simulink model "spacecraft_adcs"  (R2025b)
settings: Solver=ode4  StartTime=0.0  StopTime=600  FixedStep=0.01  RelTol=1e-3
InitFcn:
  | init_spacecraft_adcs
values from neighbouring files (symbols this model uses):
  mekf_params = struct()    [init_spacecraft_adcs.m]
undefined symbols (not defined in the file or in its folder): env, init, orbit, ref_time, sensors, sim_params, spacecraft
settings Model: Creator=cutcu  LastModifiedBy=cutcu

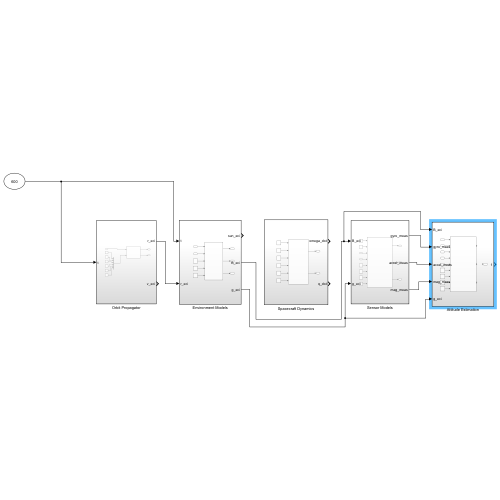
[thumbnail: Simulink's stored preview of the top-level diagram]
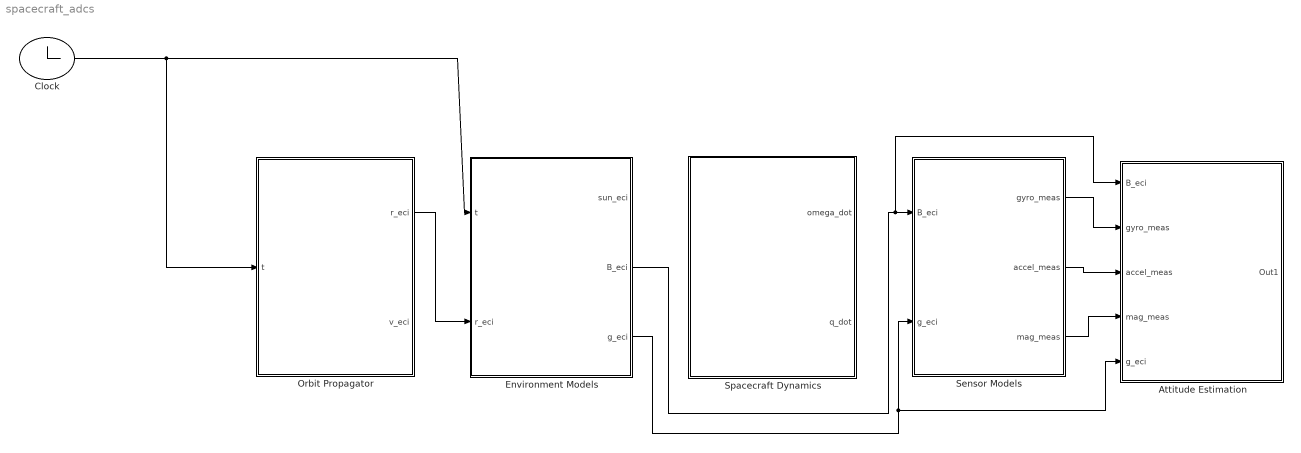
== system spacecraft_adcs ==
  Attitude Estimation : Subsystem
  Clock : Clock
  Environment Models : Subsystem
  Orbit Propagator : Subsystem
  Sensor Models : Subsystem
  Spacecraft Dynamics : Subsystem
  wires:
  Orbit Propagator/1(r_eci) -> Environment Models/2(r_eci)
  Clock/1 -> Environment Models/1(t), Orbit Propagator/1(t)
  Environment Models/3(g_eci) -> Attitude Estimation/5(g_eci), Sensor Models/2(g_eci)
  Environment Models/2(B_eci) -> Attitude Estimation/1(B_eci), Sensor Models/1(B_eci)
  Sensor Models/1(gyro_meas) -> Attitude Estimation/2(gyro_meas)
  Sensor Models/2(accel_meas) -> Attitude Estimation/3(accel_meas)
  Sensor Models/3(mag_meas) -> Attitude Estimation/4(mag_meas)

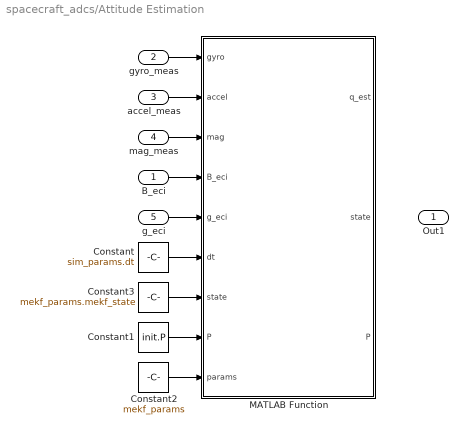
== system spacecraft_adcs/Attitude Estimation ==
  B_eci : Inport
  gyro_meas : Inport  Port=2
  accel_meas : Inport  Port=3
  mag_meas : Inport  Port=4
  g_eci : Inport  Port=5
  Constant : Constant  Value=sim_params.dt
  Constant1 : Constant  Value=init.P
  Constant2 : Constant  Value=mekf_params
  Constant3 : Constant  Value=mekf_params.mekf_state
  MATLAB Function : MATLAB Function  TreatAsAtomicUnit=on
  Out1 : Outport
  wires:
  gyro_meas/1 -> MATLAB Function/1(gyro)
  accel_meas/1 -> MATLAB Function/2(accel)
  mag_meas/1 -> MATLAB Function/3(mag)
  Constant/1 -> MATLAB Function/6(dt)
  Constant1/1 -> MATLAB Function/8("P ")
  Constant2/1 -> MATLAB Function/9(params)
  Constant3/1 -> MATLAB Function/7("state ")
  g_eci/1 -> MATLAB Function/5(g_eci)
  B_eci/1 -> MATLAB Function/4(B_eci)

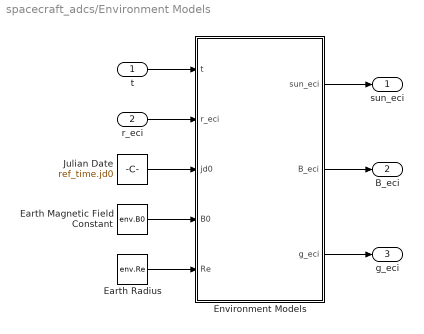
== system spacecraft_adcs/Environment Models ==
  t : Inport
  r_eci : Inport  Port=2
  Earth Magnetic Field Constant : Constant  Value=env.B0
  Earth Radius : Constant  Value=env.Re
  Environment Models : MATLAB Function  TreatAsAtomicUnit=on
  Julian Date : Constant  Value=ref_time.jd0
  sun_eci : Outport
  B_eci : Outport  Port=2
  g_eci : Outport  Port=3
  wires:
  r_eci/1 -> Environment Models/2(r_eci)
  Julian Date/1 -> Environment Models/3(jd0)
  Earth Magnetic Field Constant/1 -> Environment Models/4(B0)
  Earth Radius/1 -> Environment Models/5(Re)
  Environment Models/1(sun_eci) -> sun_eci/1
  Environment Models/2(B_eci) -> B_eci/1
  Environment Models/3(g_eci) -> g_eci/1
  t/1 -> Environment Models/1(t)

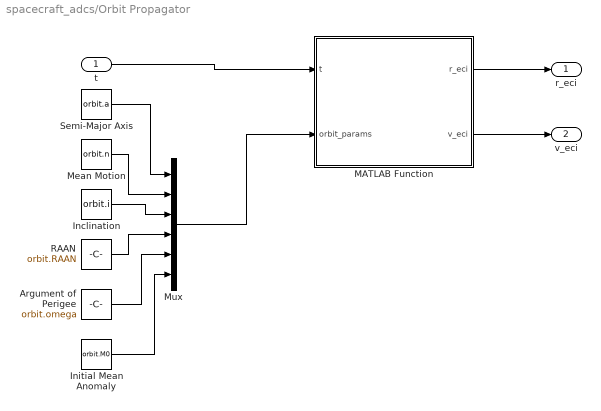
== system spacecraft_adcs/Orbit Propagator ==
  t : Inport
  Argument of Perigee : Constant  Value=orbit.omega
  Inclination : Constant  Value=orbit.i
  Initial Mean Anomaly : Constant  Value=orbit.M0
  MATLAB Function : MATLAB Function  TreatAsAtomicUnit=on
  Mean Motion : Constant  Value=orbit.n
  Mux : Mux  Inputs=6
  RAAN : Constant  Value=orbit.RAAN
  Semi-Major Axis : Constant  Value=orbit.a
  r_eci : Outport
  v_eci : Outport  Port=2
  wires:
  MATLAB Function/2(v_eci) -> v_eci/1
  MATLAB Function/1(r_eci) -> r_eci/1
  Semi-Major Axis/1 -> Mux/1
  Mean Motion/1 -> Mux/2
  Inclination/1 -> Mux/3
  RAAN/1 -> Mux/4
  Argument of Perigee/1 -> Mux/5
  Initial Mean Anomaly/1 -> Mux/6
  Mux/1 -> MATLAB Function/2(orbit_params)
  t/1 -> MATLAB Function/1(t)

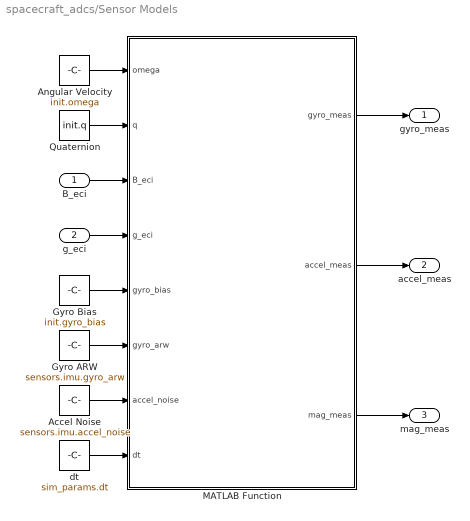
== system spacecraft_adcs/Sensor Models ==
  B_eci : Inport
  g_eci : Inport  Port=2
  Accel Noise : Constant  Value=sensors.imu.accel_noise
  Angular Velocity : Constant  Value=init.omega
  Gyro ARW : Constant  Value=sensors.imu.gyro_arw
  Gyro Bias : Constant  Value=init.gyro_bias
  MATLAB Function : MATLAB Function  TreatAsAtomicUnit=on
  Quaternion : Constant  Value=init.q
  dt : Constant  Value=sim_params.dt
  gyro_meas : Outport
  accel_meas : Outport  Port=2
  mag_meas : Outport  Port=3
  wires:
  dt/1 -> MATLAB Function/8(dt)
  B_eci/1 -> MATLAB Function/3(B_eci)
  g_eci/1 -> MATLAB Function/4(g_eci)
  Gyro ARW/1 -> MATLAB Function/6(gyro_arw)
  Accel Noise/1 -> MATLAB Function/7(accel_noise)
  Gyro Bias/1 -> MATLAB Function/5(gyro_bias)
  Quaternion/1 -> MATLAB Function/2(q)
  Angular Velocity/1 -> MATLAB Function/1(omega)
  MATLAB Function/1(gyro_meas) -> gyro_meas/1
  MATLAB Function/2(accel_meas) -> accel_meas/1
  MATLAB Function/3(mag_meas) -> mag_meas/1

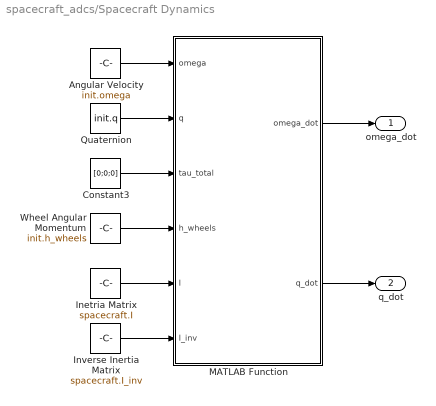
== system spacecraft_adcs/Spacecraft Dynamics ==
  Angular Velocity : Constant  Value=init.omega
  Constant3 : Constant  Value=[0;0;0]
  Inetria Matrix : Constant  Value=spacecraft.I
  Inverse Inertia Matrix : Constant  Value=spacecraft.I_inv
  MATLAB Function : MATLAB Function  TreatAsAtomicUnit=on
  Quaternion : Constant  Value=init.q
  Wheel Angular Momentum : Constant  Value=init.h_wheels
  omega_dot : Outport
  q_dot : Outport  Port=2
  wires:
  Angular Velocity/1 -> MATLAB Function/1(omega)
  Inverse Inertia Matrix/1 -> MATLAB Function/6(I_inv)
  Inetria Matrix/1 -> MATLAB Function/5(I)
  Wheel Angular Momentum/1 -> MATLAB Function/4(h_wheels)
  Quaternion/1 -> MATLAB Function/2(q)
  MATLAB Function/1(omega_dot) -> omega_dot/1
  MATLAB Function/2(q_dot) -> q_dot/1
  Constant3/1 -> MATLAB Function/3(tau_total)

== matlab function spacecraft_adcs/Environment Models/Environment Models ==
  data: t input; sun_eci output; r_eci input; jd0 input; B0 input; B_eci output; g_eci output; Re input
function [sun_eci, B_eci, g_eci] = environment_models(t, r_eci, jd0, B0, Re)
    % Sun position (simplified almanac)
    JD = jd0 + t/86400;
    T = (JD - 2451545) / 36525;
    L = mod(280.46 + 36000.77*T, 360);
    M = mod(357.53 + 35999.05*T, 360) * pi/180;
    lambda = (L + 1.915*sin(M)) * pi/180;
    eps = 23.439 * pi/180;
    sun_eci = [cos(lambda); cos(eps)*sin(lambda); sin(eps)*sin(lambda)];
    sun_eci = sun_eci / norm(sun_eci);
    
    % Magnetic field (dipole model)
    r_mag = norm(r_eci);
    r_hat = r_eci / r_mag;
    m_hat = [0; 0; 1];  % Magnetic dipole along Z
    B_eci = B0 * (Re/r_mag)^3 * (3*dot(m_hat,r_hat)*r_hat - m_hat);
    
    % Gravity direction
    g_eci = -r_eci / norm(r_eci);
end

== matlab function spacecraft_adcs/Orbit Propagator/MATLAB Function ==
  data: t input; r_eci output; orbit_params input; v_eci output
function [r_eci, v_eci] = fcn(t, orbit_params)
%#codegen
% orbit_params = [a; n; inc; RAAN; omega; M0] (6x1 vector)

    a         = orbit_params(1);
    n         = orbit_params(2);
    inc       = orbit_params(3);
    RAAN      = orbit_params(4);
    omega_arg = orbit_params(5);
    M0        = orbit_params(6);
    
    % Mean anomaly
    M = n * t + M0;
    nu = M;
    
    % Position in perifocal
    r_peri = a * [cos(nu); sin(nu); 0];
    
    % Velocity
    mu = 3.986004418e14;
    v_mag = sqrt(mu / a);
    v_peri = v_mag * [-sin(nu); cos(nu); 0];
    
    % Rotation matrix
    c_O = cos(RAAN); s_O = sin(RAAN);
    c_i = cos(inc);  s_i = sin(inc);
    c_w = cos(omega_arg); s_w = sin(omega_arg);
    
    R = [c_O*c_w - s_O*c_i*s_w,  -c_O*s_w - s_O*c_i*c_w,  s_O*s_i;
         s_O*c_w + c_O*c_i*s_w,  -s_O*s_w + c_O*c_i*c_w, -c_O*s_i;
         s_i*s_w,                 s_i*c_w,                 c_i];
    
    r_eci = R * r_peri;
    v_eci = R * v_peri;
end

== matlab function spacecraft_adcs/Spacecraft Dynamics/MATLAB Function ==
  data: omega input; omega_dot output; q input; tau_total input; h_wheels input; I input; I_inv input; q_dot output
function [omega_dot, q_dot] = spacecraft_dynamics(omega, q, tau_total, h_wheels, I, I_inv)
    % Euler's equation: I*omega_dot + omega x (I*omega + h_w) = tau
    L = I * omega + h_wheels;
    omega_dot = I_inv * (tau_total - cross(omega, L));
    
    % Quaternion kinematics: q_dot = 0.5 * Omega(omega) * q
    Omega = [0, omega(3), -omega(2), omega(1);
            -omega(3), 0, omega(1), omega(2);
             omega(2), -omega(1), 0, omega(3);
            -omega(1), -omega(2), -omega(3), 0];
    q_dot = 0.5 * Omega * q;
end

== matlab function spacecraft_adcs/Sensor Models/MATLAB Function ==
  data: omega input; gyro_meas output; q input; B_eci input; g_eci input; gyro_bias input; gyro_arw input; accel_noise input; dt input; accel_meas output; mag_meas output
function [gyro_meas, accel_meas, mag_meas] = sensor_models(omega, q, B_eci, g_eci, gyro_bias, gyro_arw, accel_noise,  dt)
    % DCM from ECI to Body
    A = quat2dcm(q);
    
    % Gyroscope (with bias and noise)
    gyro_noise = gyro_arw * sqrt(1/dt) * randn(3,1);
    gyro_meas = omega + gyro_bias + gyro_noise;
    
    % Accelerometer (gravity in body frame + noise)
    g_body = A * g_eci;
    accel_noise = accel_noise * randn(3,1);
    accel_meas = -g_body * 9.81 + accel_noise;
    
    % Magnetometer (B field in body frame + noise)
    B_body = A * B_eci;
    mag_noise = 10e-9 * randn(3,1);  % 10 nT noise
    mag_meas = B_body + mag_noise;
end

function A = quat2dcm(q)
    q1=q(1); q2=q(2); q3=q(3); q4=q(4);
    A = [q4^2+q1^2-q2^2-q3^2, 2*(q1*q2+q3*q4), 2*(q1*q3-q2*q4);
         2*(q1*q2-q3*q4), q4^2-q1^2+q2^2-q3^2, 2*(q2*q3+q1*q4);
         2*(q1*q3+q2*q4), 2*(q2*q3-q1*q4), q4^2-q1^2-q2^2+q3^2];
end

== matlab function spacecraft_adcs/Attitude Estimation/MATLAB Function ==
  data: gyro input; q_est output; accel input; mag input; B_eci input; g_eci input; dt input; state input; P input; params input; state output; P output
% Multiplicative Extended Kalman Filter (MEKF) for Attitude Estimation
% 
% IMU (gyro + accelerometer) ve Magnetometer füzyonu ile yönelim kestirimi.
% Quaternion hata temsili kullanılır (multiplicative error quaternion).
%
% Referanslar:
%   - Wertz Chapter 12, 17 - Attitude Determination and Prediction
%   - Markley (2003), "Attitude Error Representations for Kalman Filtering"
%   - Crassidis & Junkins (2012), "Optimal Estimation of Dynamic Systems"
%   - Lefferts et al. (1982), "Kalman Filtering for Spacecraft Attitude Estimation"

% State Vector (7x1 represented as 6x1 error state):
%   x = [δθ(3x1); b_gyro(3x1)]
%   δθ: attitude error (Gibbs vector / Rodrigues parameters)
%   b_gyro: gyro bias
%
% True State:
%   q_true = δq ⊗ q_est  (quaternion multiplication)
%   ω_true = ω_meas - b_gyro

% Fonksiyon çağrısı:
%   [q_est, state, P] = mekf_attitude(gyro, accel, mag, B_ref, g_ref, dt, state, P, params)
%
% Girdiler:
%   gyro    - gyro ölçümü [ωx, ωy, ωz] (rad/s) [3x1]
%   accel   - accelerometer ölçümü [ax, ay, az] (m/s^2) [3x1]
%   mag     - magnetometer ölçümü [Bx, By, Bz] (body frame) [3x1]
%   B_ref   - referans manyetik alan (ECI frame, normalize) [3x1]
%   g_ref   - referans gravity vektörü (ECI frame, normalize) [3x1]
%   dt      - zaman adımı (s)
%   state   - filtre durumu (struct)
%   P       - kovaryans matrisi [6x6]
%   params  - filtre parametreleri (struct)
%
% Çıktılar:
%   q_est   - kestirilen quaternion [q1,q2,q3,q4] [4x1]
%   state   - güncellenmiş filtre durumu
%   P       - güncellenmiş kovaryans matrisi

function [q_est, state, P] = mekf_attitude(gyro, accel, mag, B_eci, g_eci, dt, state, P, params)

B_ref = B_eci(:,k) / norm(B_eci(:,k));
g_ref = g_eci(:,k);

% Varsayılan parametreler
if nargin < 9 || isempty(params)
    params = mekf_default_params();
end

% Durumu başlat (ilk çağrıda)
if nargin < 7 || isempty(state)
    state = mekf_init_state(accel, mag, B_ref, g_ref);
end

% Kovaryansı başlat (ilk çağrıda)
if nargin < 8 || isempty(P)
    P = mekf_init_covariance(params);
end

% Girdileri sütun vektörüne çevir
gyro = gyro(:);
accel = accel(:);
mag = mag(:);
B_ref = B_ref(:);
g_ref = g_ref(:);

%% ==================== PREDICTION STEP ====================
% Gyro ölçümü ile quaternion propagasyonu

% Bias-corrected angular velocity
omega = gyro - state.gyro_bias;

% Quaternion kinematic equation (Wertz Eq. 17-2)
% q_dot = 0.5 * Omega(ω) * q
q_pred = quaternion_propagate(state.q, omega, dt);

% State transition matrix F (6x6)
% Attitude error dynamics + gyro bias dynamics
F = compute_F_matrix(omega, dt, params);

% Process noise covariance Q
Q = compute_Q_matrix(dt, params);

% Covariance prediction
P_pred = F * P * F' + Q;

%% ==================== UPDATE STEP ====================
% Magnetometer ve Accelerometer ölçümleri ile güncelleme

% Normalize ölçümler
accel_norm = accel / norm(accel);
mag_norm = mag / norm(mag);
B_ref_norm = B_ref / norm(B_ref);
g_ref_norm = g_ref / norm(g_ref);

% Predicted measurements (body frame'de beklenen vektörler)
R_pred = quaternion_to_dcm(q_pred);  % ECI -> Body DCM
g_pred = R_pred * g_ref_norm;        % Predicted gravity in body
B_pred = R_pred * B_ref_norm;        % Predicted mag field in body

% Measurement residual (innovation)
% z = [accel_meas - accel_pred; mag_meas - mag_pred]
z = [accel_norm - g_pred;
     mag_norm - B_pred];

% Measurement matrix H (6x6)
H = compute_H_matrix(g_pred, B_pred);

% Measurement noise covariance R (6x6)
R = compute_R_matrix(params);

% Kalman gain
S = H * P_pred * H' + R;
K = P_pred * H' / S;

% State update
dx = K * z;  % [δθ(3x1); δb(3x1)]

% Quaternion update (multiplicative)
delta_theta = dx(1:3);
delta_q = error_to_quaternion(delta_theta);
q_est = quaternion_multiply(delta_q, q_pred);
q_est = q_est / norm(q_est);  % Normalize

% Gyro bias update
state.gyro_bias = state.gyro_bias + dx(4:6);

% Covariance update (Joseph form for numerical stability)
I_KH = eye(6) - K * H;
P = I_KH * P_pred * I_KH' + K * R * K';

% Durumu güncelle
state.q = q_est;

end


%% ==================== HELPER FUNCTIONS ====================

function state = mekf_init_state(accel, mag, B_ref, g_ref)
% TRIAD ile başlangıç yönelimi hesapla
    accel = accel(:) / norm(accel);
    mag = mag(:) / norm(mag);
    B_ref = B_ref(:) / norm(B_ref);
    g_ref = g_ref(:) / norm(g_ref);
    
    % TRIAD: gravity daha doğru, mag daha az doğru
    [q_init, ~] = triad_algorithm(accel, mag, g_ref, B_ref);
    
    state.q = q_init;
    state.gyro_bias = zeros(3,1);
end


function P = mekf_init_covariance(params)
% Başlangıç kovaryans matrisi
    P = diag([params.init_attitude_var * ones(1,3), ...
              params.init_bias_var * ones(1,3)]);
end


function params = mekf_default_params()
% MEKF varsayılan parametreleri
    
    % Process noise (gyro)
    params.gyro_noise = 0.15 * (pi/180) / sqrt(3600);  % ARW: 0.15 deg/sqrt(h)
    params.gyro_bias_noise = 0.5 * (pi/180) / 3600;    % Bias instability: 0.5 deg/h
    
    % Measurement noise
    params.accel_noise = 0.01;   % g (normalized) - çok hassas değil
    params.mag_noise = 0.05;     % normalized - daha gürültülü
    
    % Initial covariance
    params.init_attitude_var = (10 * pi/180)^2;  % 10 deg initial uncertainty
    params.init_bias_var = (1 * pi/180 / 3600)^2;  % 1 deg/h initial bias uncertainty
end


function F = compute_F_matrix(omega, dt, params)
% State transition matrix (discrete time)
% F = exp(F_c * dt) ≈ I + F_c * dt for small dt
    
    % Skew-symmetric matrix of omega
    omega_cross = skew(omega);
    
    % Continuous time F matrix
    % [δθ_dot]   [-ω×   -I] [δθ  ]
    % [b_dot ] = [0      0] [b   ]
    F_c = [-omega_cross, -eye(3);
           zeros(3,3),   zeros(3,3)];
    
    % Discrete time approximation
    F = eye(6) + F_c * dt;
end


function Q = compute_Q_matrix(dt, params)
% Process noise covariance matrix
    
    % Gyro noise affects attitude
    Q_theta = (params.gyro_noise^2 * dt) * eye(3);
    
    % Gyro bias random walk
    Q_bias = (params.gyro_bias_noise^2 * dt) * eye(3);
    
    Q = blkdiag(Q_theta, Q_bias);
end


function H = compute_H_matrix(g_pred, B_pred)
% Measurement Jacobian matrix
% h(x) = R(q) * v_ref
% dh/dδθ = -[R*v_ref]× = -[v_body_pred]×
    
    H_accel = -skew(g_pred);
    H_mag = -skew(B_pred);
    
    % Bias'ın ölçüm üzerinde direkt etkisi yok
    H = [H_accel, zeros(3,3);
         H_mag,   zeros(3,3)];
end


function R = compute_R_matrix(params)
% Measurement noise covariance matrix
    R_accel = params.accel_noise^2 * eye(3);
    R_mag = params.mag_noise^2 * eye(3);
    
    R = blkdiag(R_accel, R_mag);
end


function q_new = quaternion_propagate(q, omega, dt)
% Quaternion propagation using angular velocity
% q_dot = 0.5 * Omega(ω) * q
    
    % Omega matrix
    wx = omega(1); wy = omega(2); wz = omega(3);
    Omega = [0,   wz, -wy,  wx;
            -wz,  0,   wx,  wy;
             wy, -wx,  0,   wz;
            -wx, -wy, -wz,  0];
    
    % First-order integration (good for small dt)
    q_dot = 0.5 * Omega * q;
    q_new = q + q_dot * dt;
    q_new = q_new / norm(q_new);
end


function A = quaternion_to_dcm(q)
% Quaternion'dan DCM'e dönüşüm
    q1 = q(1); q2 = q(2); q3 = q(3); q4 = q(4);
    
    A = [q1^2-q2^2-q3^2+q4^2,   2*(q1*q2+q3*q4),       2*(q1*q3-q2*q4);
         2*(q1*q2-q3*q4),       -q1^2+q2^2-q3^2+q4^2,  2*(q2*q3+q1*q4);
         2*(q1*q3+q2*q4),       2*(q2*q3-q1*q4),       -q1^2-q2^2+q3^2+q4^2];
end


function q = error_to_quaternion(delta_theta)
% Küçük açı hatasından quaternion'a dönüşüm
% δq ≈ [δθ/2; 1] for small δθ
    
    delta_theta = delta_theta(:);
    norm_dt = norm(delta_theta);
    
    if norm_dt < 1e-10
        q = [0; 0; 0; 1];
    else
        q = [delta_theta/2; 1];
        q = q / norm(q);
    end
end


function q = quaternion_multiply(p, q)
% Quaternion multiplication: r = p ⊗ q
    p1 = p(1); p2 = p(2); p3 = p(3); p4 = p(4);
    q1 = q(1); q2 = q(2); q3 = q(3); q4 = q(4);
    
    r = [p4*q1 + p1*q4 + p2*q3 - p3*q2;
         p4*q2 - p1*q3 + p2*q4 + p3*q1;
         p4*q3 + p1*q2 - p2*q1 + p3*q4;
         p4*q4 - p1*q1 - p2*q2 - p3*q3];
    q = r;
end


function S = skew(v)
% Skew-symmetric (cross product) matrix
    S = [0,    -v(3),  v(2);
         v(3),  0,    -v(1);
        -v(2),  v(1),  0];
end
